simulink model "simulink_drone_ekf"  (R2024b)
settings: Solver=VariableStepAuto  StartTime=0.0  StopTime=10.0  RelTol=1e-3
values from neighbouring files (symbols this model uses):
  barometer_sample_time = 1/100    (= 0.01)    [simulink_vars.m]
  barometer_variance = [0.0625]    [simulink_vars.m]
  gps_sample_time = 1/20    (= 0.05)    [simulink_vars.m]
  gps_variance = 0.0025 * ones(1,3)    [simulink_vars.m]
  imu_drift = [0.0,0.0,0.0,0.00,0.00,0.00,0.0,0.0,0.0]    [simulink_vars.m]
  imu_sample_time = 1/100    (= 0.01)    [simulink_vars.m]
  imu_variance = [0.01,0.01,0.01,0.01,0.01,0.01,0.01,0.01,0.01]    [offline_kalman_kinematic.m]    (also in simulink_vars.m = [0.029,0.029,0.029,0.1225,0.1225,0.1225,0.0037,0.0037,0.0037)
undefined symbols (not defined in the file or in its folder): barometer_noise
libraries: sharedTrackingLibrary x1
settings Model: Creator=dp271  LastModifiedBy=dp271

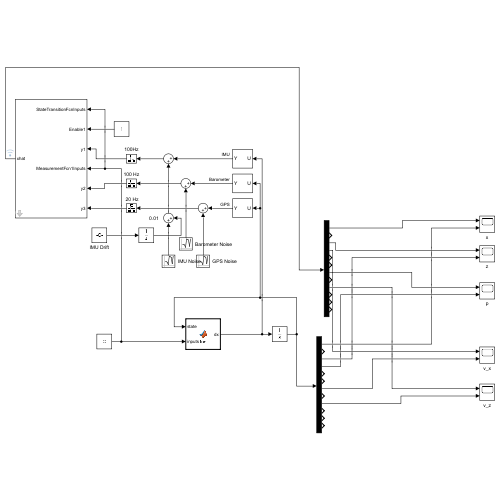
[thumbnail: Simulink's stored preview of the top-level diagram]
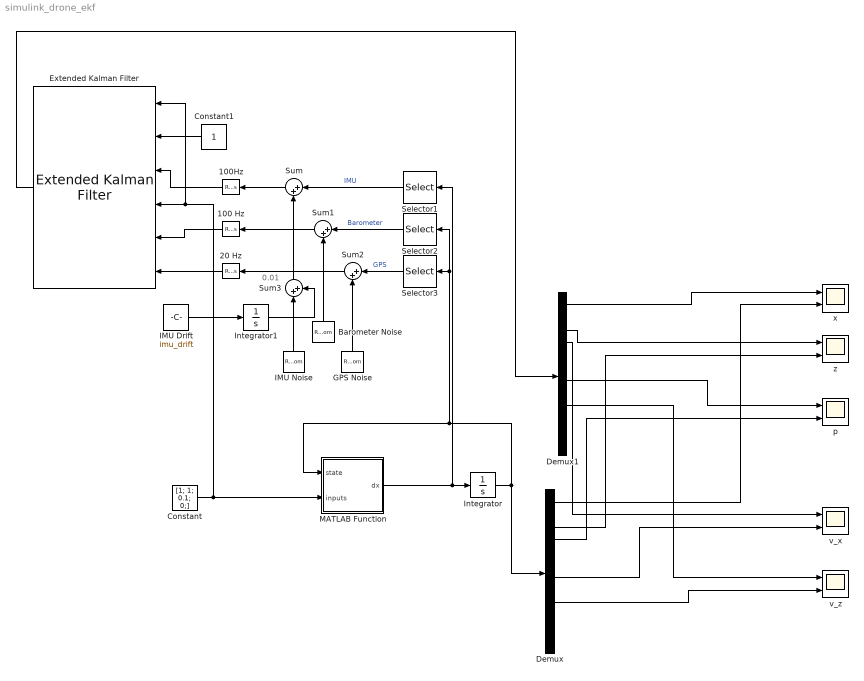
== system simulink_drone_ekf ==
  note: 0.01
  " 20 Hz" : RateTransition  OutPortSampleTime=gps_sample_time
  100 Hz : RateTransition  OutPortSampleTime=barometer_sample_time
  100Hz : RateTransition  OutPortSampleTime=imu_sample_time
  Barometer Noise : RandomNumber  Variance=barometer_noise  SampleTime=barometer_sample_time
  Constant : Constant  Value=[1; 1; 0.1; 0;]
  Constant1 : Constant  VectorParams1D=off
  Demux : Demux  Outputs=12
  Demux1 : Demux  Outputs=12
  Extended Kalman Filter : sharedTrackingLibrary/Extended Kalman Filter  StateTransitionFcn=drone_step  HasStateTransitionJacobianFcn=off  HasAdditiveProcessNoise=Additive  ProcessNoise=process_noise  HasTimeVaryingProcessNoise=off  HasStateTransitionFcnExtraArgument=1  InitialState=zeros(12,1)  InitialStateCovariance=initial_noise  MeasurementFcn1=imu  HasMeasurementJacobianFcn1=off  HasMeasurementEnablePort1=on  HasAdditiveMeasurementNoise1=Additive  MeasurementNoise1=diag(imu_variance)  HasTimeVaryingMeasurementNoise1=off  HasMeasurementFcnExtraArgument1=1  HasMeasurementWrapping1=off  MeasurementFcn2=barometer  HasMeasurementJacobianFcn2=off  HasMeasurementEnablePort2=off  HasAdditiveMeasurementNoise2=Additive  MeasurementNoise2=diag(barometer_variance)  HasTimeVaryingMeasurementNoise2=off  HasMeasurementFcnExtraArgument2=0  HasMeasurementWrapping2=off  MeasurementFcn3=gps  HasMeasurementJacobianFcn3=off  HasMeasurementEnablePort3=off  HasAdditiveMeasurementNoise3=Additive  MeasurementNoise3=diag(gps_variance)  HasTimeVaryingMeasurementNoise3=off  HasMeasurementFcnExtraArgument3=0  HasMeasurementWrapping3=off  MeasurementFcn4=myMeasurementFcn  HasMeasurementJacobianFcn4=off  HasMeasurementEnablePort4=off  HasAdditiveMeasurementNoise4=Additive  MeasurementNoise4=1  HasTimeVaryingMeasurementNoise4=off  HasMeasurementFcnExtraArgument4=0  HasMeasurementWrapping4=off  MeasurementFcn5=myMeasurementFcn  HasMeasurementJacobianFcn5=off  HasMeasurementEnablePort5=off  HasAdditiveMeasurementNoise5=Additive  MeasurementNoise5=1  HasTimeVaryingMeasurementNoise5=off  HasMeasurementFcnExtraArgument5=0  HasMeasurementWrapping5=off  EnableMultirate=on  StateTransitionFcnSampleTime=ekf_sample_time  MeasurementFcn1SampleTime=imu_sample_time  MeasurementFcn2SampleTime=barometer_sample_time  MeasurementFcn3SampleTime=gps_sample_time  MeasurementFcn4SampleTime=1  MeasurementFcn5SampleTime=1  UseCurrentEstimator=on  OutputStateCovariance=off  DataType=double  SampleTime=0.01  NumberOfMeasurements=3
  GPS Noise : RandomNumber  Mean=zeros(3,1)  Variance=gps_variance  SampleTime=gps_sample_time
  IMU Drift : Constant  Value=imu_drift
  IMU Noise : RandomNumber  Mean=zeros(9,1)  Variance=imu_variance  SampleTime=imu_sample_time
  Integrator : Integrator  InitialCondition=zeros(12,1)
  Integrator1 : Integrator  InitialCondition=zeros(9,1)
  MATLAB Function : MATLAB Function  TreatAsAtomicUnit=on
  Selector1 : Selector  IndexOptions=Index vector (dialog)  Indices=[4 5 6 7 8 9 10 11 12]  OutputSizes=1
  Selector2 : Selector  IndexOptions=Index vector (dialog)  Indices=[3]  OutputSizes=1
  Selector3 : Selector  IndexOptions=Index vector (dialog)  Indices=[1 2 3]  OutputSizes=1
  Sum{,1..3} (4 alike) : Sum  Inputs=|++
  p : Scope  NumInputPorts=2
  v_x : Scope  NumInputPorts=2
  v_z : Scope  NumInputPorts=2
  x : Scope  NumInputPorts=2
  z : Scope  NumInputPorts=2
  wires:
  MATLAB Function/1(dx) -> Selector1/1, Integrator/1
  Constant/1 -> MATLAB Function/2(inputs), Extended Kalman Filter/1, Extended Kalman Filter/4
  Demux/3 -> z/2
  Demux/1 -> x/2
  Extended Kalman Filter/1 -> Demux1/1
  Demux1/1 -> x/1
  Demux1/3 -> z/1
  100Hz/1 -> Extended Kalman Filter/3
  Integrator/1 -> Demux/1, MATLAB Function/1(state), Selector3/1, Selector2/1
  Demux/9 -> v_z/2
  Demux1/9 -> v_z/1
  100 Hz/1 -> Extended Kalman Filter/5
  " 20 Hz"/1 -> Extended Kalman Filter/6
  Demux1/4 -> p/1
  Demux/4 -> p/2
  Demux1/7 -> v_x/1
  Demux/7 -> v_x/2
  Constant1/1 -> Extended Kalman Filter/2
  Selector2/1 -> Sum1/1  "Barometer"
  Sum1/1 -> 100 Hz/1
  Selector1/1 -> Sum/1  "IMU"
  Sum/1 -> 100Hz/1
  Selector3/1 -> Sum2/1  "GPS"
  Sum2/1 -> " 20 Hz"/1
  Barometer Noise/1 -> Sum1/2
  GPS Noise/1 -> Sum2/2
  IMU Noise/1 -> Sum3/1
  Integrator1/1 -> Sum3/2
  Sum3/1 -> Sum/2
  IMU Drift/1 -> Integrator1/1

== matlab function simulink_drone_ekf/MATLAB Function ==
  data: state input; inputs input; dx output
function dx = fcn(state, inputs)

    dx = drone_dynamics(state, inputs);

end
